simulink model "receiveBPSK_PLUTOSDR"  (R2023b)
settings: Solver=VariableStepAuto  StartTime=0.0  StopTime=inf  RelTol=1e-3  EnableMultiTasking=on
values from neighbouring files (symbols this model uses):
  numSymsTot = 256    [numSymsTot.mat]
undefined symbols (not defined in the file or in its folder): Fs, ip, usb
libraries: commsync2 x2, plutoradiolib x1, commrfcorlib x1, commdigbbndpm3 x1, commfilt2 x1, simulink x1
settings Model: Creator=prust  LastModifiedBy=龚玲玉
settings SolverCC: AlgebraicLoopSolver=TrustRegion
settings DataIOCC: ReturnWorkspaceOutputs=off
settings OptimizationCC: LifeSpan=inf
settings DebuggingCC: UnconnectedInputMsg=warning  UnconnectedOutputMsg=warning  UnconnectedLineMsg=warning  SFUnexpectedBacktrackingDiag=warning  SFNoUnconditionalDefaultTransitionDiag=warning  SFExecutionAtInitializationDiag=none  ArithmeticOperatorsInVariantConditions=warning
settings ModelReferenceCC: EnableRefExpFcnMdlSchedulingChecks=on
settings SFSimCC: SimUseLocalCustomCode=off  CustomCodeUndefinedFunction=UseInterfaceOnly
settings RTWCC: RTWUseLocalCustomCode=off  DLArmComputeVersion=19.05
settings CodeAppCC: StateflowObjectComments=on
settings GRTTargetCC: TargetLangStandard=C89/C90 (ANSI)
settings ConfigComp: CovMetricSettings=dw  CovSaveCumulativeToWorkspaceVar=on  CovSaveSingleToWorkspaceVar=on  CovExternalEMLEnable=off

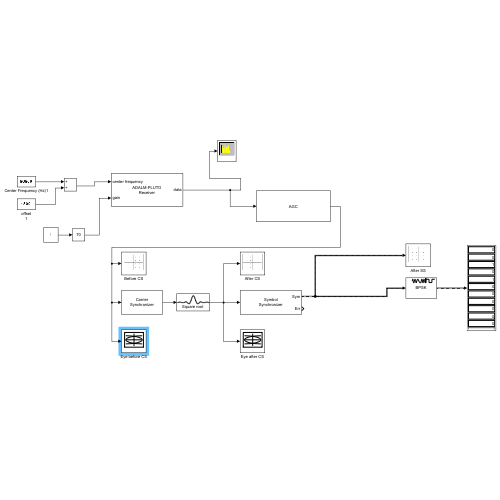
[thumbnail: Simulink's stored preview of the top-level diagram]
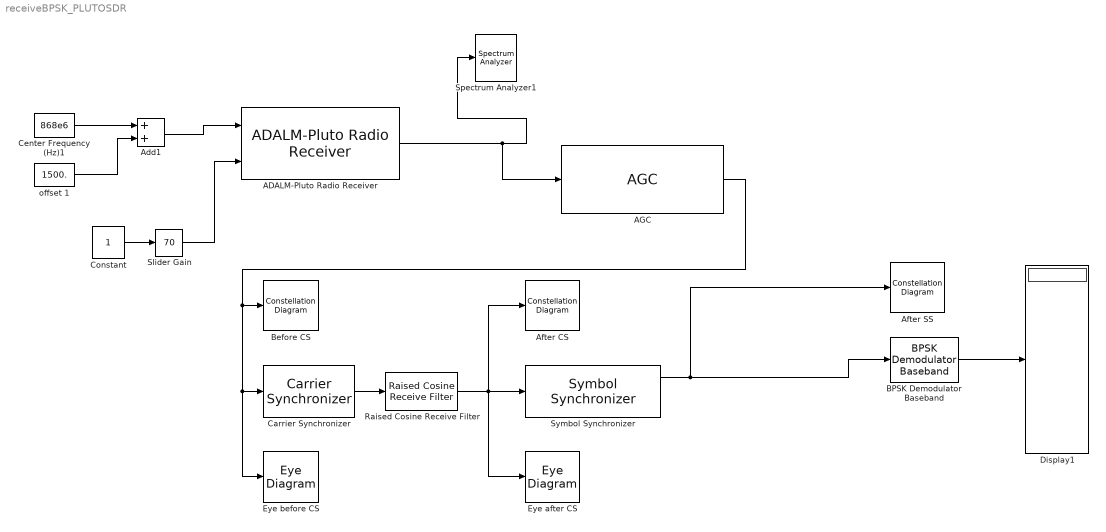
== system receiveBPSK_PLUTOSDR ==
  ADALM-Pluto Radio Receiver : plutoradiolib/ADALM-Pluto Radio Receiver  RadioID=usb:0  uri=ip:10.0.0.200  CenterFrequencySource=Input Port  CenterFrequency=2.4e9  GainSource=AGC Slow Attack  GainSourceBlock=Input Port  Gain=10  ChannelMapping=1  BasebandSampleRate=300e3  OutputDataType=single  SamplesPerFrame=numSymsTot*10*15  OverflowOutputPort=off  EnableBurstMode=off  NumFramesInBurst=1  ShowAdvancedProperties=off  UseCustomFilter=off  filtPathRates=[737280000 11520000 3840000 1920000 960000 240000]  filtCoefficients=[-192 82 85 -215 228 -102 -110 290 -318 145 160 -426 471 -215 -238 633 -697 318 349 -923 1009 -457 -498 1309 -1423 640 693 -1812 1959 -876 -945 2458 -2647 1180 1268 -3290 3534 -1572 -1688 4375 -4698 2091 2247 -5836 6284 -2807 -3031 7918 -8588 3870 4225 -11182 12324 -5662 -6330 17255 -19735 9507 11312 -33568 43355 -25227 -42139 305542 305542 -42139 -25227 43355 -33568 11312 9507 -19735 17255 -6330 -5662 12324 -11182 4225 3870 -8588 7918 -3031 -2807 6284 -5836 2247 2091 -4698 4375 -1688 -1572 3534 -3290 1268 1180 -2647 2458 -945 -876 1959 -1812 693 640 -1423 1309 -498 -457 1009 -923 349 318 -697 633 -238 -215 471 -426 160 145 -318 290 -110 -102 228 -215 85 82 -192]  filtCoefficientSize=128  filtDecimInterpFactor=4  filtGain=-12  filtRFBandwidth=18000000  filterConfigStruct=struct()  EnableQuadratureCorrection=off  EnableRFDCCorrection=off  EnableBasebandDCCorrection=on  FrequencyCorrection=0  OverrideSampleTime=off  SampleTime=0.02  DataTimeout=Inf  ENSMPinControlMode=None  BISTLoopbackMode=Disabled  BISTToneInject=Disabled  BISTSignalGen=PRBS  BISTToneFreq=Fs/32  BISTToneLevel=0
  AGC : commrfcorlib/AGC  LegacyMode=off  DetectorMethod=Rectifier  LoopMethod=Linear  UpdatePeriod=100  StepSize=0.1  AdaptationStepSize=0.1  DesiredOutputPower=0.1  AveragingLength=200  MaximumGain=30  MaxPowerGain=40  GainOutputPort=off  InputPowerOutputPort=off  SimulateUsing=Interpreted execution
  Add1 : Sum
  After CS : ConstellationDiagram  WindowPosition=[755.000000,281.000000,341.000000,346.000000,]  ScopeFrameLocation=window  SamplesPerSymbol=10  SymbolsToDisplaySource=Property  SymbolsToDisplay=100  ReferenceConstellation=BPSK  XLimits=[-1.8347 1.888]  YLimits=[-1.8347 1.888]  DefaultConfigurationName=comm.scopes.ConstellationDiagramBlockCfg
  After SS : ConstellationDiagram  WindowPosition=[930.000000,170.000000,427.000000,345.000000,]  ScopeFrameLocation=window  SamplesPerSymbol=10  SymbolsToDisplaySource=Property  SymbolsToDisplay=200  ReferenceConstellation=BPSK  XLimits=[-2.7261 2.0629]  YLimits=[-2.7261 2.0629]  MaximizeAxes=off  DefaultConfigurationName=comm.scopes.ConstellationDiagramBlockCfg
  BPSK Demodulator Baseband : commdigbbndpm3/BPSK Demodulator Baseband  DecType=Hard decision  VarSource=Dialog  Variance=1  Ph=pi  outDtype=Inherit via internal rule  derotateFactorWordLen=16  derotateFactorDataTypeStr=Inherit: Same word length as input  derotateFactorLastDataTypeStr=Inherit: Same word length as input
  Before CS : ConstellationDiagram  WindowPosition=[763.000000,285.000000,329.000000,346.000000,]  ScopeFrameLocation=window  SamplesPerSymbol=30  SymbolsToDisplaySource=Property  SymbolsToDisplay=100  ReferenceConstellation=BPSK  XLimits=[-1.5991 1.3577]  YLimits=[-1.9686 1.7273]  DefaultConfigurationName=comm.scopes.ConstellationDiagramBlockCfg
  Carrier Synchronizer : commsync2/Carrier Synchronizer  Modulation=BPSK  ModulationPhaseOffset=Auto  CustomPhaseOffset=0  SamplesPerSymbol=15  DampingFactor=0.707  NormalizedLoopBandwidth=0.01  EstimatedPhaseErrorOutputPort=off  SimulateUsing=Code generation
  Center Frequency (Hz)1 : Constant  Value=868e6
  Constant : Constant
  Display1 : Display
  Eye after CS : EyeDiagram
  Eye before CS : EyeDiagram
  Raised Cosine Receive Filter : commfilt2/Raised Cosine Receive Filter  filtType=Square root  R=0.5  filtSpan=2  N=15  downFactor=3  downOffset=0  filterGain=1  InputProcessing=Columns as channels (frame based)  RateOptions=Enforce single-rate processing  framing=Mute  checkCoeff=off  variableName=rcRxFilt1  currentFiltSpan=4  D=(4)/2  inputOffset=0  sampMode=Mute  saveAsFlag=0  rateMode=Downsampling  checkGain=Normalized  launchFVT=on  roundingMode=Floor  overflowMode=off  coeffDataTypeStr=Inherit: Same word length as input  coeffMin=[]  coeffMax=[]  coeffLastDataTypeStr=Inherit: Same word length as input  accumDataTypeStr=Inherit: Same as product output  accumLastDataTypeStr=Inherit: Same as product output  outputDataTypeStr=Inherit: Same as accumulator  outputMin=[]  outputMax=[]  outputLastDataTypeStr=Inherit: Same as accumulator
  Slider Gain : simulink/Math Operations/Slider Gain  gain=70  low=5  high=70
  Spectrum Analyzer1 : SpectrumAnalyzer  WindowPosition=[501.000000,310.000000,800.000000,450.000000,]  Visible=on  ScopeFrameLocation=window  Method=Welch  SampleRate=300000  AxesScaling=Manual  Span=300000  StartFrequency=-150000  StopFrequency=150000  AveragingMethod=Running  YLimits=[-89.367524113707403899,28.453797216119536273]  DefaultConfigurationName=spbscopes.SpectrumAnalyzerBlockCfg  IsFrequencyInputMode=0  FrequencyVectorPort=0  FrequencyVectorFromPort=0  FrequencyInputRBWPort=0  FrequencyInputRBWFromPort=0
  Symbol Synchronizer : commsync2/Symbol Synchronizer  Modulation=PAM/PSK/QAM  TimingErrorDetector=Mueller-Muller (decision-directed)  SamplesPerSymbol=5  DampingFactor=0.707  NormalizedLoopBandwidth=0.01  DetectorGain=1.0  TimingErrorOutputPort=on  SimulateUsing=Interpreted execution
  offset 1 : Constant  Value=1500.
  wires:
  AGC/1 -> Before CS/1, Eye before CS/1, Carrier Synchronizer/1
  BPSK Demodulator Baseband/1 -> Display1/1
  Constant/1 -> Slider Gain/1
  Raised Cosine Receive Filter/1 -> Symbol Synchronizer/1, Eye after CS/1, After CS/1
  Carrier Synchronizer/1 -> Raised Cosine Receive Filter/1
  Slider Gain/1 -> ADALM-Pluto Radio Receiver/2
  Symbol Synchronizer/1 -> BPSK Demodulator Baseband/1, After SS/1
  Add1/1 -> ADALM-Pluto Radio Receiver/1
  ADALM-Pluto Radio Receiver/1 -> AGC/1, Spectrum Analyzer1/1
  offset 1/1 -> Add1/2
  Center Frequency (Hz)1/1 -> Add1/1
